simulink library "LaRController_cl"  (R2022a)
settings: Solver=VariableStepAuto  StartTime=0.0  StopTime=10.0  RelTol=1e-3
undefined symbols (not defined in the file or in its folder): el, elevSet, env, FLIGHTCONTROLLER, fltCtrl, initializeBussesFromBlock, thr, vhcl, wnch
libraries: simulink x1, filteredPIDControllerAW_ul x1, filteredPIDControllerAWGS_ul x1, ctrlAllocMatrix3Comp_cl x1, eulAng2RotMat_ul x1, angleBtw2Vecs_ul x1, vrlib x1, alphaBeta_ul x1, filteredPIDController_ul x1, gnd2TanRotation_ul x1
settings Model: Creator=jldanie5  LastModifiedBy=lhill8
settings SolverCC: AlgebraicLoopSolver=TrustRegion
settings DataIOCC: ReturnWorkspaceOutputs=off
settings DebuggingCC: UnconnectedInputMsg=warning  UnconnectedOutputMsg=warning  UnconnectedLineMsg=warning  SFMachineParentedDataDiag=warning  ArithmeticOperatorsInVariantConditions=warning
settings SFSimCC: CustomCodeUndefinedFunction=UseInterfaceOnly

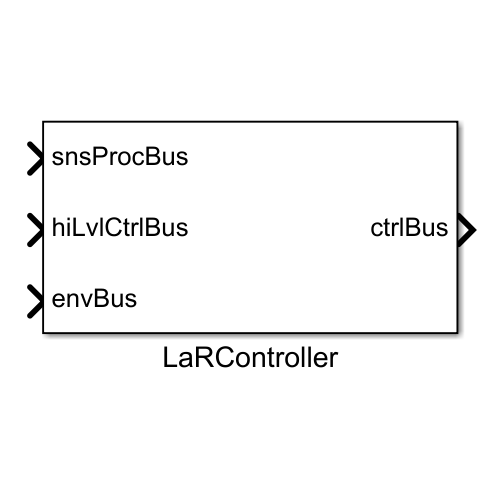
[thumbnail: Simulink's stored preview of the top-level diagram]
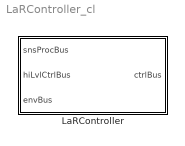
== system LaRController_cl ==
  LaRController : Subsystem  LoadFcn=initializeBussesFromBlock(gcb)  InitFcn=initializeBussesFromBlock(gcb)  StartFcn=initializeBussesFromBlock(gcb)  VariantControl=strcmpi(FLIGHTCONTROLLER,'LaRController')  mask{initPosForInitSStar=vhcl.initPosVecGnd.Value, fluidDensity=env.water.density.Value, LaRCtrl=fltCtrl, aeroStruct=vhcl.struct('OCT.aeroSurf'), LaRThr=thr.tether1, LaRWnch=wnch.winch1}
      mask prompts: initPosForInitSStar "Initial Position"; fluidDensity "Fluid Density"; LaRCtrl "Controller"; aeroStruct "Aerodynamic Structure"; LaRThr "Tether"; LaRWnch "Winch"
      settings: MinAlgLoopOccurrences=on
      mask DialogControl Container3 Prompt: courseFollow Params
      mask DialogControl Container4 Prompt: setpointToOutput Params

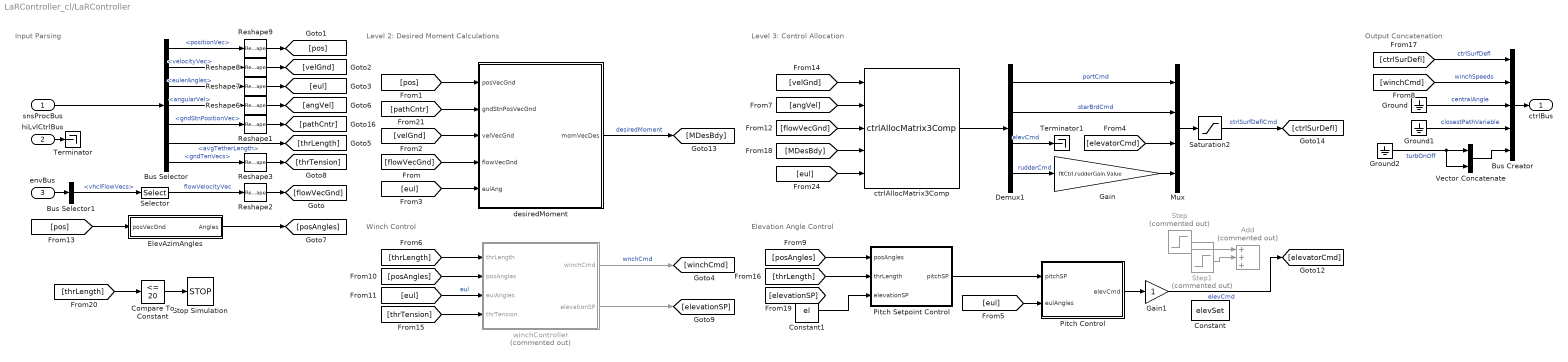
== system LaRController_cl/LaRController ==
  note: Winch Control
  note: Level 3: Control Allocation
  note: Output Concatenation
  note: Level 2: Desired Moment Calculations
  note: Input Parsing
  note: Elevation Angle Control
  snsProcBus : Inport  OutDataTypeStr=Bus: sensorsProcessingBus
  hiLvlCtrlBus : Inport  Port=2  OutDataTypeStr=Bus: hiLvlCtrlBus
  envBus : Inport  Port=3  OutDataTypeStr=Bus: envBus
  Add : Sum  Commented=on  Inputs=+++
  Bus Creator : BusCreator  Inputs=5  OutDataTypeStr=Bus: fltCtrlBus
      settings: InheritFromInputs=off
  Bus Selector : BusSelector  OutputSignals=positionVec,velocityVec,eulerAngles,angularVel,gndStnPositionVec,avgTetherLength,gndTenVecs
  Bus Selector1 : BusSelector  OutputSignals=vhclFlowVecs
  Compare To Constant : simulink/Logic and Bit Operations/Compare To Constant  relop=<=  const=20  OutDataTypeStr=boolean
  Constant : Constant  Value=elevSet
  Constant1 : Constant  Value=el
  Demux1 : Demux
  ElevAzimAngles : Subsystem
  Gain : Gain  Gain=fltCtrl.rudderGain.Value
  Gain1 : Gain
  Ground : Ground
  Ground1 : Ground
  Ground2 : Ground
  Mux : Mux
  Pitch Control : Subsystem
  Pitch Setpoint Control : Subsystem
  Reshape{1..3,6..9} (7 alike) : Reshape  OutputDimensionality=Column vector (2-D)
  Saturation2 : Saturate  UpperLimit=LaRCtrl.controlSigMax.upperLimit.Value  LowerLimit=LaRCtrl.controlSigMax.lowerLimit.Value
  Selector : Selector  NumberOfDimensions=2  InputPortWidth=3  IndexOptions=Select all,Index vector (dialog)  Indices=[1 3],5  OutputSizes=1,1
  Step : Step  Commented=on  Time=200  After=0  SampleTime=0
  Step1 : Step  Commented=on  Time=210  After=0  SampleTime=0
  Stop Simulation : Stop
  Terminator : Terminator
  Terminator1 : Terminator
  Vector Concatenate : Concatenate
  ctrlAllocMatrix3Comp : ctrlAllocMatrix3Comp_cl/ctrlAllocMatrix3Comp  aeroStruct=vhcl.struct('OCT.aeroSurf')  fluidDensity=fluidDensity  arms=vhcl.struct('OCT.thrAttch')
  desiredMoment : Subsystem
  winchController : Subsystem  Commented=on  mask{thrC=LaRThr, ctrlC=LaRCtrl}
      mask prompts: thrC "Tether:"; ctrlC "Controller:"
  ctrlBus : Outport  OutDataTypeStr=Bus: fltCtrlBus  VectorParamsAs1DForOutWhenUnconnected=off
  wires:
  snsProcBus/1 -> Bus Selector/1
  Bus Selector/2 -> Reshape8/1  "<velocityVec>"
  Bus Selector/1 -> Reshape9/1  "<positionVec>"
  Bus Selector/3 -> Reshape7/1  "<eulerAngles>"
  Bus Creator/1 -> ctrlBus/1
  [winchCmd] -> Bus Creator/2  "winchSpeeds"
  Ground/1 -> Bus Creator/3  "centralAngle"
  Ground1/1 -> Bus Creator/4  "closestPathVariable"
  desiredMoment/1(momVecDes) -> [MDesBdy]  "desiredMoment"
  Bus Selector/4 -> Reshape6/1  "<angularVel>"
  [angVel] -> ctrlAllocMatrix3Comp/2
  [velGnd] -> ctrlAllocMatrix3Comp/1
  [flowVecGnd] -> ctrlAllocMatrix3Comp/3
  Demux1/1 -> Mux/1  "portCmd"
  Demux1/2 -> Mux/2  "starBrdCmd"
  ctrlAllocMatrix3Comp/1 -> Demux1/1
  [MDesBdy] -> ctrlAllocMatrix3Comp/4
  [ctrlSurDefl] -> Bus Creator/1  "ctrlSurfDefl"
  Saturation2/1 -> [ctrlSurDefl]  "ctrlSurfDeflCmd"
  Reshape2/1 -> [flowVecGnd]
  Reshape6/1 -> [angVel]
  Reshape7/1 -> [eul]
  Reshape8/1 -> [velGnd]
  Reshape9/1 -> [pos]
  [eul] -> ctrlAllocMatrix3Comp/5
  Selector/1 -> Reshape2/1  "flowVelocityVec"
  envBus/1 -> Bus Selector1/1
  Bus Selector1/1 -> Selector/1  "<vhclFlowVecs>"
  Reshape1/1 -> [pathCntr]
  Bus Selector/5 -> Reshape1/1  "<gndStnPositionVec>"
  [pos] -> desiredMoment/1(posVecGnd)
  [pathCntr] -> desiredMoment/2(gndStnPosVecGnd)
  [velGnd] -> desiredMoment/3(velVecGnd)
  [eul] -> desiredMoment/5(eulAng)
  [flowVecGnd] -> desiredMoment/4(flowVecGnd)
  Gain/1 -> Mux/4
  Demux1/4 -> Gain/1  "rudderCmd"
  hiLvlCtrlBus/1 -> Terminator/1
  Mux/1 -> Saturation2/1
  Demux1/3 -> Terminator1/1  "elevCmd"
  [elevatorCmd] -> Mux/3
  Bus Selector/6 -> [thrLength]  "<avgTetherLength>"
  [thrLength] -> winchController/1(thrLength)
  winchController/1(winchCmd) -> [winchCmd]  "wnchCmd"
  [eul] -> Pitch Control/2(eulAngles)
  Pitch Control/1(elevCmd) -> Gain1/1
  [posAngles] -> Pitch Setpoint Control/1(posAngles)
  Pitch Setpoint Control/1(pitchSP) -> Pitch Control/1(pitchSP)
  Gain1/1 -> [elevatorCmd]  "elevCmd"
  [posAngles] -> winchController/2(posAngles)
  [eul] -> winchController/3(eulAngles)  "eul"
  Ground2/1 -> Vector Concatenate/2, Vector Concatenate/1  "turbOnOff"
  [pos] -> ElevAzimAngles/1(posVecGnd)
  ElevAzimAngles/1(Angles) -> [posAngles]
  Bus Selector/7 -> Reshape3/1  "<gndTenVecs>"
  [thrTension] -> winchController/4(thrTension)
  Reshape3/1 -> [thrTension]
  [thrLength] -> Pitch Setpoint Control/2(thrLength)
  winchController/2(elevationSP) -> [elevationSP]
  [thrLength] -> Compare To Constant/1
  Compare To Constant/1 -> Stop Simulation/1
  Step/1 -> Add/1
  Step1/1 -> Add/2
  Vector Concatenate/1 -> Bus Creator/5
  Constant1/1 -> Pitch Setpoint Control/3(elevationSP)

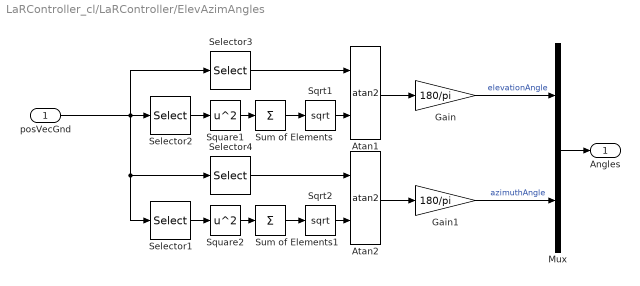
== system LaRController_cl/LaRController/ElevAzimAngles ==
  posVecGnd : Inport
  Atan1 : Trigonometry  Operator=atan2
  Atan2 : Trigonometry  Operator=atan2
  Gain : Gain  Gain=180/pi
  Gain1 : Gain  Gain=180/pi
  Mux : Mux  Inputs=2
  Selector1 : Selector  InputPortWidth=3  IndexOptions=Index vector (dialog)  Indices=1  OutputSizes=1
  Selector2 : Selector  InputPortWidth=3  IndexOptions=Index vector (dialog)  Indices=[1 2]  OutputSizes=1
  Selector3 : Selector  InputPortWidth=3  IndexOptions=Index vector (dialog)  Indices=3  OutputSizes=1
  Selector4 : Selector  InputPortWidth=3  IndexOptions=Index vector (dialog)  Indices=2  OutputSizes=1
  Sqrt1 : Sqrt
  Sqrt2 : Sqrt
  Square1 : Math  Operator=square  SignedPower=on
  Square2 : Math  Operator=square  SignedPower=on
  Sum of Elements : Sum  Inputs=+
  Sum of Elements1 : Sum  Inputs=+
  Angles : Outport
  wires:
  Sqrt1/1 -> Atan1/2
  Square1/1 -> Sum of Elements/1
  Selector3/1 -> Atan1/1
  Sum of Elements/1 -> Sqrt1/1
  Atan1/1 -> Gain/1
  Selector2/1 -> Square1/1
  Selector4/1 -> Atan2/1
  Selector1/1 -> Square2/1
  Sum of Elements1/1 -> Sqrt2/1
  posVecGnd/1 -> Selector3/1, Selector4/1, Selector1/1, Selector2/1
  Atan2/1 -> Gain1/1
  Sqrt2/1 -> Atan2/2
  Square2/1 -> Sum of Elements1/1
  Gain/1 -> Mux/1  "elevationAngle"
  Gain1/1 -> Mux/2  "azimuthAngle"
  Mux/1 -> Angles/1

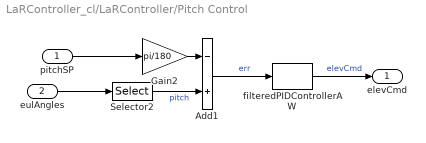
== system LaRController_cl/LaRController/Pitch Control ==
  pitchSP : Inport
  eulAngles : Inport  Port=2
  Add1 : Sum  Inputs=-+
  Gain2 : Gain  Gain=pi/180
  Selector2 : Selector  InputPortWidth=3  IndexOptions=Index vector (dialog)  Indices=2  OutputSizes=1
  filteredPIDControllerAW : filteredPIDControllerAW_ul/filteredPIDControllerAW  kp=LaRCtrl.elevCmd.kp.Value  ki=LaRCtrl.elevCmd.ki.Value  kd=LaRCtrl.elevCmd.kd.Value  tau=LaRCtrl.elevCmd.tau.Value  cmax=LaRCtrl.controlSigMax.upperLimit.Value  cmin=LaRCtrl.controlSigMax.lowerLimit.Value
  elevCmd : Outport
  wires:
  Selector2/1 -> Add1/2  "pitch"
  filteredPIDControllerAW/1 -> elevCmd/1  "elevCmd"
  pitchSP/1 -> Gain2/1
  eulAngles/1 -> Selector2/1
  Gain2/1 -> Add1/1
  Add1/1 -> filteredPIDControllerAW/1  "err"

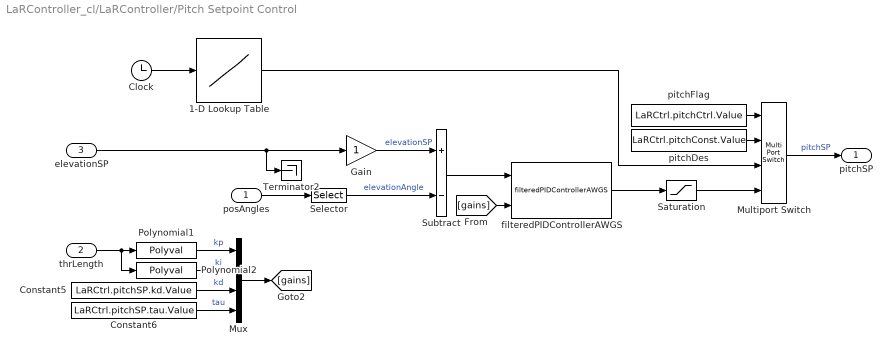
== system LaRController_cl/LaRController/Pitch Setpoint Control ==
  posAngles : Inport
  thrLength : Inport  Port=2
  elevationSP : Inport  Port=3
  1-D Lookup Table : Lookup_n-D  NumberOfTableDimensions=1  BreakpointsForDimension1=LaRCtrl.pitchTime.Value  Table=LaRCtrl.pitchLookup.Value  InterpMethod=Flat  InternalRulePriority=Speed  RndMeth=Simplest
  Clock : Clock
  Constant5 : Constant  Value=LaRCtrl.pitchSP.kd.Value
  Constant6 : Constant  Value=LaRCtrl.pitchSP.tau.Value
  Gain : Gain
  Multiport Switch : MultiPortSwitch  DataPortOrder=Specify indices  Inputs=2  DataPortIndices={0,1,2}  SaturateOnIntegerOverflow=off  InputSameDT=off
  Mux : Mux
  Polynomial1 : Polyval  Coefs=[LaRCtrl.pitchSPkpSlope.Value LaRCtrl.pitchSPkpInt.Value]
  Polynomial2 : Polyval  Coefs=[LaRCtrl.pitchSPkiSlope.Value LaRCtrl.pitchSPkiInt.Value]
  Saturation : Saturate  UpperLimit=LaRCtrl.pitchAngleMax.upperLimit.Value  LowerLimit=LaRCtrl.pitchAngleMax.lowerLimit.Value
  Selector : Selector  InputPortWidth=2  IndexOptions=Index vector (dialog)  Indices=1  OutputSizes=1
  Subtract : Sum  Inputs=+-
  Terminator2 : Terminator
  filteredPIDControllerAWGS : filteredPIDControllerAWGS_ul/filteredPIDControllerAWGS  cmax=LaRCtrl.pitchAngleMax.upperLimit.Value  cmin=LaRCtrl.pitchAngleMax.lowerLimit.Value
  pitchDes : Constant  Value=LaRCtrl.pitchConst.Value
  pitchFlag : Constant  Value=LaRCtrl.pitchCtrl.Value
  pitchSP : Outport
  wires:
  pitchFlag/1 -> Multiport Switch/1
  Multiport Switch/1 -> pitchSP/1  "pitchSP"
  pitchDes/1 -> Multiport Switch/2
  posAngles/1 -> Selector/1
  Clock/1 -> 1-D Lookup Table/1
  Selector/1 -> Subtract/2  "elevationAngle"
  Gain/1 -> Subtract/1  "elevationSP"
  1-D Lookup Table/1 -> Multiport Switch/3
  elevationSP/1 -> Gain/1, Terminator2/1
  Subtract/1 -> filteredPIDControllerAWGS/1
  Polynomial1/1 -> Mux/1  "kp"
  Polynomial2/1 -> Mux/2  "ki"
  Constant5/1 -> Mux/3  "kd"
  Constant6/1 -> Mux/4  "tau"
  [gains] -> filteredPIDControllerAWGS/2
  Mux/1 -> [gains]
  thrLength/1 -> Polynomial2/1, Polynomial1/1
  filteredPIDControllerAWGS/1 -> Saturation/1
  Saturation/1 -> Multiport Switch/4

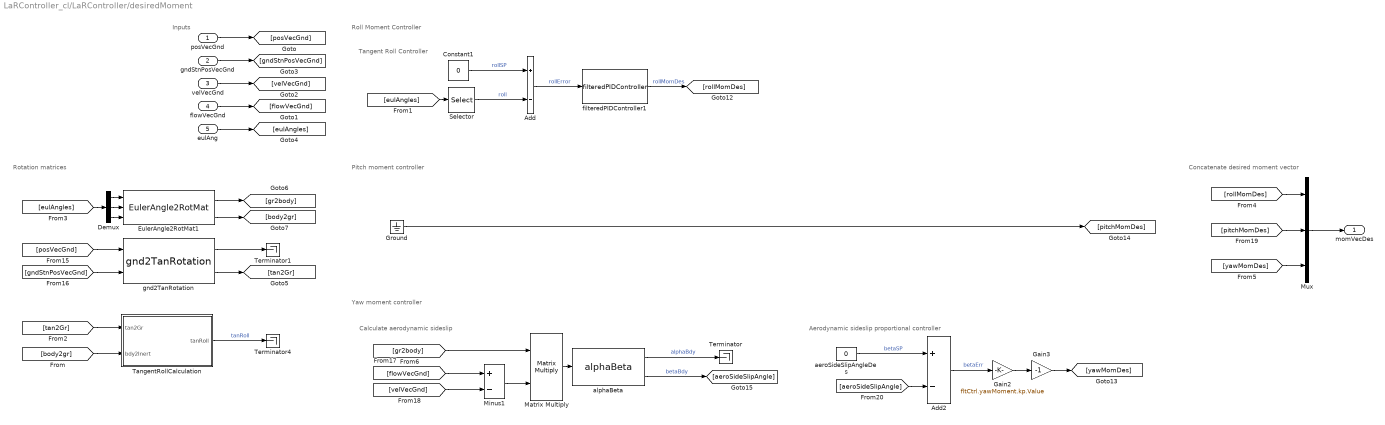
== system LaRController_cl/LaRController/desiredMoment ==
  note: Inputs
  note: Rotation matrices
  note: Tangent Roll Controller
  note: Concatenate desired moment vector
  note: Aerodynamic sideslip proportional controller
  note: Calculate aerodynamic sideslip
  note: Yaw moment controller
  note: Pitch moment controller
  note: Roll Moment Controller
  posVecGnd : Inport
  gndStnPosVecGnd : Inport  Port=2
  velVecGnd : Inport  Port=3
  flowVecGnd : Inport  Port=4
  eulAng : Inport  Port=5
  Add : Sum  Inputs=+-
  Add2 : Sum  Inputs=+-
  Constant1 : Constant  Value=0
  Demux : Demux  Outputs=3
  EulerAngle2RotMat1 : eulAng2RotMat_ul/EulerAngle2RotMat  SystemSampleTime=-1  VariantActivationTime=update diagram  Latency=0  AutoFrameSizeCalculation=off
  Gain2 : Gain  Gain=fltCtrl.yawMoment.kp.Value
  Gain3 : Gain  Gain=-1
  Ground : Ground
  Matrix Multiply : Product  Multiplication=Matrix(*)
  Minus1 : Sum  Inputs=+-
  Mux : Mux  Inputs=3
  Selector : Selector  InputPortWidth=3  IndexOptions=Index vector (dialog)  Indices=1  OutputSizes=1
  TangentRollCalculation : Subsystem
  Terminator : Terminator
  Terminator1 : Terminator
  Terminator4 : Terminator
  aeroSideSlipAngleDes : Constant  Value=0
  alphaBeta : alphaBeta_ul/alphaBeta  SystemSampleTime=-1  VariantActivationTime=update diagram  Latency=0  AutoFrameSizeCalculation=off
  filteredPIDController1 : filteredPIDController_ul/filteredPIDController  kp=LaRCtrl.rollMoment.kp.Value  ki=0  kd=LaRCtrl.rollMoment.kd.Value  Value=LaRCtrl.rollMoment.tau.Value  externalReset=none
  gnd2TanRotation : gnd2TanRotation_ul/gnd2TanRotation  SystemSampleTime=-1  VariantActivationTime=update diagram  Latency=0  AutoFrameSizeCalculation=off
  momVecDes : Outport  VectorParamsAs1DForOutWhenUnconnected=off
  wires:
  [aeroSideSlipAngle] -> Add2/2
  [yawMomDes] -> Mux/3
  [rollMomDes] -> Mux/1
  gnd2TanRotation/1 -> Terminator1/1
  gnd2TanRotation/2 -> [tan2Gr]
  [gndStnPosVecGnd] -> gnd2TanRotation/2
  [posVecGnd] -> gnd2TanRotation/1
  Constant1/1 -> Add/1  "rollSP"
  gndStnPosVecGnd/1 -> [gndStnPosVecGnd]
  [pitchMomDes] -> Mux/2
  alphaBeta/1 -> Terminator/1  "alphaBdy"
  Gain3/1 -> [yawMomDes]
  Mux/1 -> momVecDes/1
  aeroSideSlipAngleDes/1 -> Add2/1  "betaSP"
  Add2/1 -> Gain2/1  "betaErr"
  alphaBeta/2 -> [aeroSideSlipAngle]  "betaBdy"
  Matrix Multiply/1 -> alphaBeta/1
  [gr2body] -> Matrix Multiply/1
  EulerAngle2RotMat1/1 -> [gr2body]
  EulerAngle2RotMat1/2 -> [body2gr]
  Demux/2 -> EulerAngle2RotMat1/2
  Demux/1 -> EulerAngle2RotMat1/1
  Demux/3 -> EulerAngle2RotMat1/3
  [flowVecGnd] -> Minus1/1
  [velVecGnd] -> Minus1/2
  Minus1/1 -> Matrix Multiply/2
  Gain2/1 -> Gain3/1
  filteredPIDController1/1 -> [rollMomDes]  "rollMomDes"
  flowVecGnd/1 -> [flowVecGnd]
  Add/1 -> filteredPIDController1/1  "rollError"
  velVecGnd/1 -> [velVecGnd]
  posVecGnd/1 -> [posVecGnd]
  eulAng/1 -> [eulAngles]
  [eulAngles] -> Demux/1
  [eulAngles] -> Selector/1
  Selector/1 -> Add/2  "roll"
  Ground/1 -> [pitchMomDes]
  TangentRollCalculation/1(tanRoll) -> Terminator4/1  "tanRoll"
  [tan2Gr] -> TangentRollCalculation/1(tan2Gr)
  [body2gr] -> TangentRollCalculation/2(bdy2Inert)

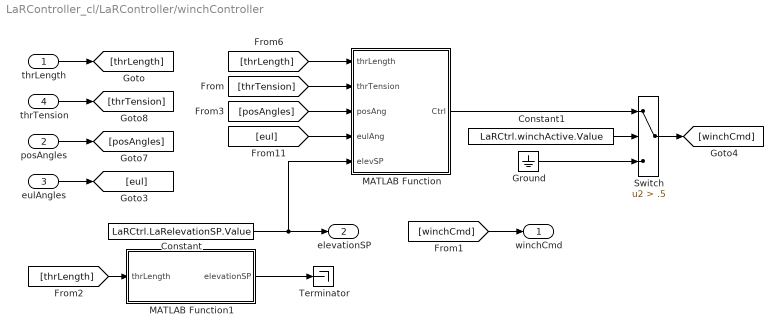
== system LaRController_cl/LaRController/winchController ==
  thrLength : Inport
  posAngles : Inport  Port=2
  eulAngles : Inport  Port=3
  thrTension : Inport  Port=4
  Constant : Constant  Value=LaRCtrl.LaRelevationSP.Value
  Constant1 : Constant  Value=LaRCtrl.winchActive.Value
  Ground : Ground
  MATLAB Function : MATLAB Function  TreatAsAtomicUnit=on  mask{leash=LaRCtrl.shortLeashLength.Value, spd=LaRCtrl.nomSpoolSpeed.Value, coneWidth=LaRCtrl.LaRelevationSPErr.Value}
      mask prompts: leash "Short Leash Length [m]"; spd "Nominal Spool Speed [m/s]"; coneWidth "Elevation Angle Error Threshold"
  MATLAB Function1 : MATLAB Function  TreatAsAtomicUnit=on  mask{elevSP1=LaRCtrl.LaRelevationSP.Value, elevSP2=50}
      mask prompts: elevSP1 "Nominal Elevation Setpoint [deg]"; elevSP2 "Final Elevation Setpoint [deg]"
  Switch : Switch  Criteria=u2 > Threshold  Threshold=.5  SaturateOnIntegerOverflow=off  InputSameDT=off
  Terminator : Terminator
  winchCmd : Outport
  elevationSP : Outport  Port=2
  wires:
  thrLength/1 -> [thrLength]
  posAngles/1 -> [posAngles]
  [winchCmd] -> winchCmd/1
  eulAngles/1 -> [eul]
  [eul] -> MATLAB Function/4(eulAng)
  [posAngles] -> MATLAB Function/3(posAng)
  [thrLength] -> MATLAB Function/1(thrLength)
  thrTension/1 -> [thrTension]
  [thrTension] -> MATLAB Function/2(thrTension)
  [thrLength] -> MATLAB Function1/1(thrLength)
  Constant/1 -> MATLAB Function/5(elevSP), elevationSP/1
  MATLAB Function1/1(elevationSP) -> Terminator/1
  Switch/1 -> [winchCmd]
  Ground/1 -> Switch/3
  Constant1/1 -> Switch/2
  MATLAB Function/1(Ctrl) -> Switch/1

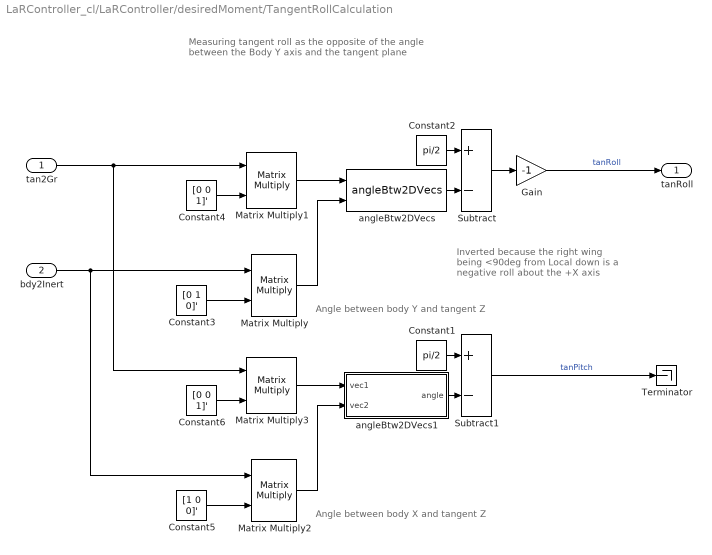
== system LaRController_cl/LaRController/desiredMoment/TangentRollCalculation ==
  note: Measuring tangent roll as the opposite
      | of the angle between the Body Y axis
      | and the tangent plane
  note: Angle between body Y and tangent Z
  note: Inverted because the right wing
      | being <90deg from Local down
      | is a negative roll about the +X axis
  note: Angle between body X and tangent Z
  tan2Gr : Inport
  bdy2Inert : Inport  Port=2
  Constant1 : Constant  Value=pi/2
  Constant2 : Constant  Value=pi/2
  Constant3 : Constant  Value=[0 1 0]'
  Constant4 : Constant  Value=[0 0 1]'
  Constant5 : Constant  Value=[1 0 0]'
  Constant6 : Constant  Value=[0 0 1]'
  Gain : Gain  Gain=-1
  Matrix Multiply{,1..3} (4 alike) : Product  Multiplication=Matrix(*)
  Subtract : Sum  Inputs=+-
  Subtract1 : Sum  Inputs=+-
  Terminator : Terminator
  angleBtw2DVecs : angleBtw2Vecs_ul/angleBtw2DVecs  SystemSampleTime=-1  Latency=0  AutoFrameSizeCalculation=off
  angleBtw2DVecs1 : Subsystem
  tanRoll : Outport  VectorParamsAs1DForOutWhenUnconnected=off
  wires:
  Constant3/1 -> Matrix Multiply/2
  angleBtw2DVecs/1 -> Subtract/2
  Constant2/1 -> Subtract/1
  Matrix Multiply1/1 -> angleBtw2DVecs/1
  Constant4/1 -> Matrix Multiply1/2
  Matrix Multiply/1 -> angleBtw2DVecs/2
  Subtract/1 -> Gain/1
  Gain/1 -> tanRoll/1  "tanRoll"
  bdy2Inert/1 -> Matrix Multiply2/1, Matrix Multiply/1
  Subtract1/1 -> Terminator/1  "tanPitch"
  tan2Gr/1 -> Matrix Multiply3/1, Matrix Multiply1/1
  Matrix Multiply2/1 -> angleBtw2DVecs1/2(vec2)
  Constant6/1 -> Matrix Multiply3/2
  Matrix Multiply3/1 -> angleBtw2DVecs1/1(vec1)
  Constant1/1 -> Subtract1/1
  angleBtw2DVecs1/1(angle) -> Subtract1/2
  Constant5/1 -> Matrix Multiply2/2

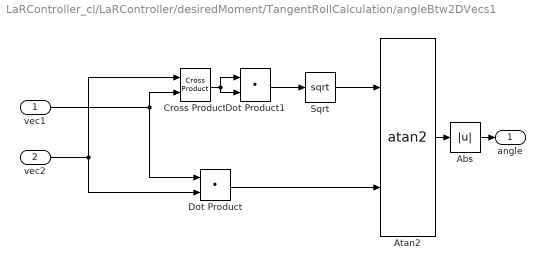
== system LaRController_cl/LaRController/desiredMoment/TangentRollCalculation/angleBtw2DVecs1 ==
  vec1 : Inport
  vec2 : Inport  Port=2
  Abs : Abs  SaturateOnIntegerOverflow=off
  Atan2 : Trigonometry  Operator=atan2
  Cross Product : vrlib/Utilities/Cross Product
  Dot Product : DotProduct  OutDataTypeStr=Inherit: Inherit via internal rule
  Dot Product1 : DotProduct  OutDataTypeStr=Inherit: Inherit via internal rule
  Sqrt : Sqrt
  angle : Outport  VectorParamsAs1DForOutWhenUnconnected=off
  wires:
  Atan2/1 -> Abs/1
  vec1/1 -> Dot Product/1, Cross Product/2
  vec2/1 -> Cross Product/1, Dot Product/2
  Cross Product/1 -> Dot Product1/1, Dot Product1/2
  Dot Product/1 -> Atan2/2
  Abs/1 -> angle/1
  Dot Product1/1 -> Sqrt/1
  Sqrt/1 -> Atan2/1

== matlab function LaRController_cl/LaRController/winchController/MATLAB Function1 ==
  data: thrLength input; elevationSP output; elevSP1 parameter; elevSP2 parameter
function elevationSP = fcn(thrLength,elevSP1, elevSP2)

if thrLength > 95
    elevationSP = elevSP1;
else
    elevationSP = elevSP2;
end

== matlab function LaRController_cl/LaRController/winchController/MATLAB Function ==
  data: thrLength input; thrTension input; posAng input; Ctrl output; eulAng input; coneWidth parameter; leash parameter; spd parameter; elevSP input
function Ctrl  = fcn(thrLength, thrTension, posAng, eulAng, coneWidth, leash, spd, elevSP)

roll = eulAng(1)*180/pi;                                %   deg - Roll angle 
% pitch = eulAng(2)*180/pi;                               %   deg - Pitch angle 
% yaw = eulAng(3)*180/pi;                                 %   deg - Yaw angle 

elevationAngle = posAng(1);                             %   deg - Elevation angle 
elevationError = abs(elevSP-elevationAngle);            %   deg - Elevation angle error 
% if thrLength < 100
%     spd = spd;
% end
nomWidth = coneWidth/2;                                 %   deg - Width of elevation cone where nominal speed is allowed
x = [nomWidth coneWidth];
y = [-spd 0];
m = (y(2)-y(1))/(x(2)-x(1));

thrErr = thrLength-leash;                               %   m - Tether length error 

if thrErr < 1
    gain = 0.01*thrErr+0.5;
else
    gain = 1;
end

if abs(roll) > 2.5
    Ctrl = 0;
elseif elevationError <= coneWidth
    if thrErr > 1
        Ctrl = max(min(m*(elevationError-x(1))+y(1),0),-spd*gain);
    else
        Ctrl = 0;
    end
else
    Ctrl = 0;
end
